simulink model "Dinamica6DOF"  (R2026a)
settings: Solver=FixedStepAuto  StopTime=C.Tfim  FixedStep=0.01  MaxStep=0.001
values from neighbouring files (symbols this model uses):
  C = CondLanc6DOF    [VooUnico6DOF.m]
  cte_grav = 9.8    [CondLanc6DOF.m]    (also in DadosMissil.m; VooUnico6DOF.m; plot6DOF.m)
  D = DadosCGInerciaComum(D)    [DadosCGInercia.m]    (also in PlotGMax.m = DadosCGInercia(D); VooUnico6DOF.m = DadosCGInercia(D))
  dados =     [M_aed.mat]
  M_CD = [8.341 8.24 8.141 8.043 7.946 7.851 7.76 7.674 7.595 7.523 7.46 7.4 ... (1365 elements, 21x5x13)]    [M_aed.mat]
  M_CM = [42.757 43.119 43.498 43.905 44.357 44.839 45.319 45.775 46.191 46.536 46.769 46.963 ... (1365 elements, 21x5x13)]    [M_aed.mat]
  M_CMQ = [-1543.746 -1552.906 -1559.915 -1565.64 -1570.662 -1573.443 -1572.931 -1569.859 -1564.198 -1553.449 -1535.22 -1514.504 ... (1365 elements, 21x5x13)]    [M_aed.mat]
  M_CN = [-21.126 -21.088 -21.046 -20.997 -20.94 -20.877 -20.812 -20.749 -20.692 -20.644 -20.613 -20.587 ... (1365 elements, 21x5x13)]    [M_aed.mat]
  R2D = 180/pi    (= 57.2957795131)    [VooUnico6DOF.m]    (also in plot6DOF.m)
undefined symbols (not defined in the file or in its folder): Newton, Raphson
libraries: aerolibasang x4, sharedutil x2, shared6dof x2, aerolibatmos2 x1, dspmtrx3 x1
settings Model: Creator=carlberto-old  LastModifiedBy=Savio
settings SolverCC: AlgebraicLoopSolver=LineSearch

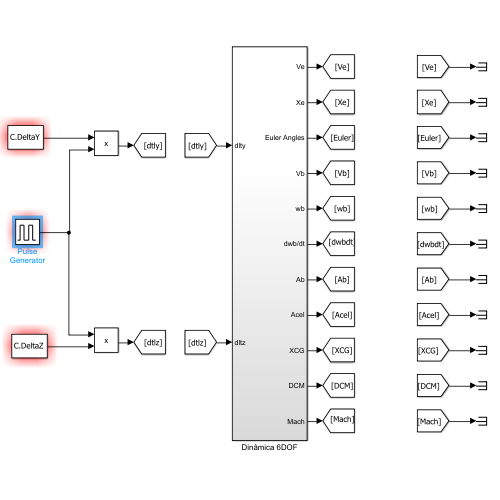
[thumbnail: Simulink's stored preview of the top-level diagram]
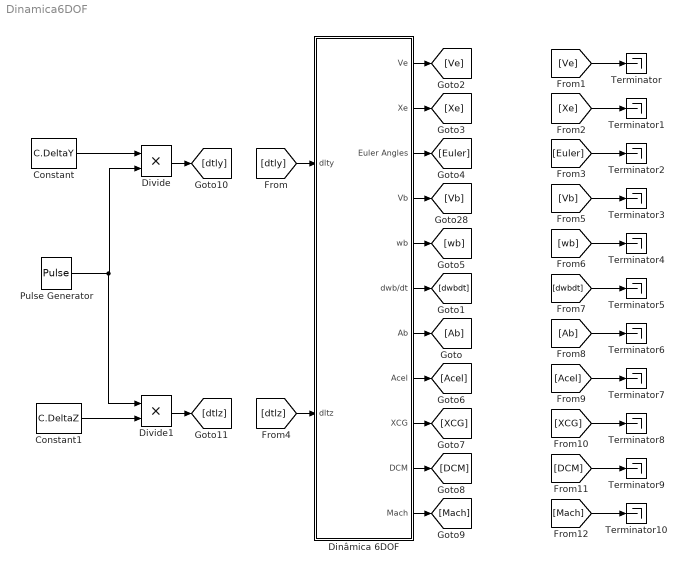
== system Dinamica6DOF ==
  Constant : Constant  Value=C.DeltaY
  Constant1 : Constant  Value=C.DeltaZ
  Dinâmica 6DOF : Subsystem
  Divide : Product  Inputs=**
  Divide1 : Product  Inputs=**
  Pulse Generator : DiscretePulseGenerator  PulseType=Time based  Period=C.Tfim/4  PulseWidth=50  PhaseDelay=D.TTrav
  Terminator{,1..10} (11 alike) : Terminator
  wires:
  Dinâmica 6DOF/2(Xe) -> [Xe]
  Dinâmica 6DOF/3(Euler Angles) -> [Euler]
  Dinâmica 6DOF/5(wb) -> [wb]
  Dinâmica 6DOF/1(Ve) -> [Ve]
  Dinâmica 6DOF/7(Ab) -> [Ab]
  Dinâmica 6DOF/6(dwb/dt) -> [dwbdt]
  Dinâmica 6DOF/4(Vb) -> [Vb]
  Dinâmica 6DOF/10(DCM) -> [DCM]
  Dinâmica 6DOF/9(XCG) -> [XCG]
  Dinâmica 6DOF/8(Acel) -> [Acel]
  Dinâmica 6DOF/11(Mach) -> [Mach]
  [dtlz] -> Dinâmica 6DOF/2(dltz)
  [dtly] -> Dinâmica 6DOF/1(dlty)
  [Ve] -> Terminator/1
  [Xe] -> Terminator1/1
  [Euler] -> Terminator2/1
  [Vb] -> Terminator3/1
  [wb] -> Terminator4/1
  [dwbdt] -> Terminator5/1
  [Ab] -> Terminator6/1
  [Acel] -> Terminator7/1
  [XCG] -> Terminator8/1
  [DCM] -> Terminator9/1
  [Mach] -> Terminator10/1
  Divide/1 -> [dtly]
  Constant/1 -> Divide/1
  Pulse Generator/1 -> Divide1/1, Divide/2
  Divide1/1 -> [dtlz]
  Constant1/1 -> Divide1/2

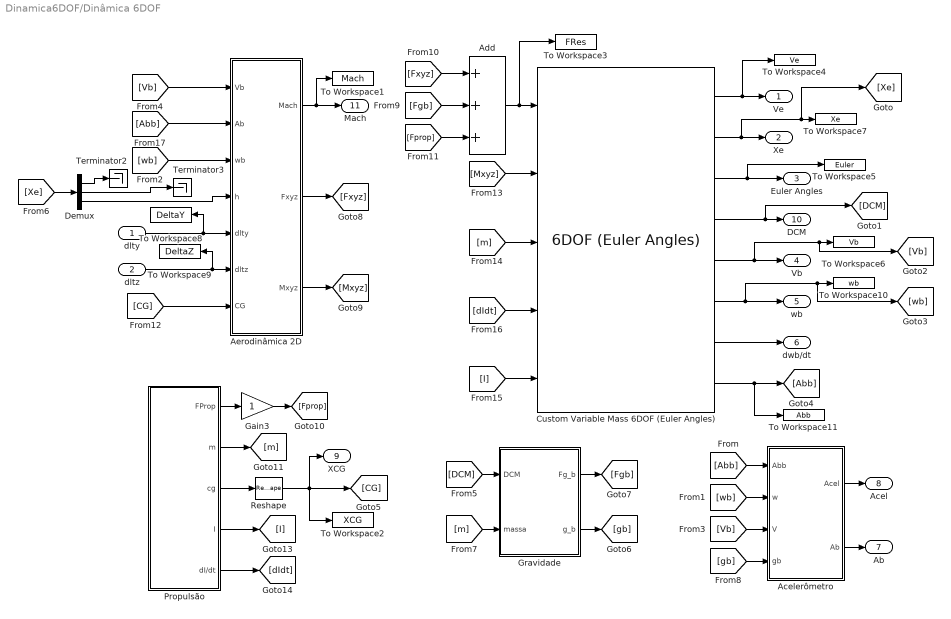
== system Dinamica6DOF/Dinâmica 6DOF ==
  dlty : Inport
  dltz : Inport  Port=2
  Acelerômetro : Subsystem
  Add : Sum  Inputs=+++
  Aerodinâmica 2D : Subsystem
  Custom Variable Mass 6DOF (Euler Angles) : shared6dof/6DOF (Euler Angles)  units=Metric (MKS)  mtype=Custom Variable  rep=Euler Angles  xme_0=[C.Xm0 C.Ym0 -C.Zm0]  Vm_0="[C.Vmx0  C.Vmy0   C.Vmz0]"  eul_0="[C.Phim0  C.Tetam0   C.Psim0]"  pm_0=[C.p0 C.q0 C.r0]  mass_0=1.0  mass_e=0.5  mass_f=2.0  inertia=eye(3)  inertia_e=eye(3)  inertia_f=2*eye(3)  k_quat=1.0  vre_flag=off  abi_flag=off  aMode=aMode  xme_statename=''  Vm_statename=''  eul_statename=''  quat_statename=''  pm_statename=''  mass_statename=''
  Demux : Demux  Outputs=3
  Gain3 : Gain
  Gravidade : Subsystem
  Propulsão : Subsystem
  Reshape : Reshape
  Terminator2 : Terminator
  Terminator3 : Terminator
  To Workspace1 : ToWorkspace  VariableName=Mach  SaveFormat=Timeseries  SampleTime=-1
  To Workspace10 : ToWorkspace  VariableName=wb  SaveFormat=Timeseries  SampleTime=-1
  To Workspace11 : ToWorkspace  VariableName=Abb  SaveFormat=Timeseries  SampleTime=-1
  To Workspace2 : ToWorkspace  VariableName=XCG  SaveFormat=Timeseries  SampleTime=-1
  To Workspace3 : ToWorkspace  VariableName=FRes  SaveFormat=Timeseries  SampleTime=-1
  To Workspace4 : ToWorkspace  VariableName=Ve  SaveFormat=Timeseries  SampleTime=-1
  To Workspace5 : ToWorkspace  VariableName=Euler  SaveFormat=Timeseries  SampleTime=-1
  To Workspace6 : ToWorkspace  VariableName=Vb  SaveFormat=Timeseries  SampleTime=-1
  To Workspace7 : ToWorkspace  VariableName=Xe  SaveFormat=Timeseries  SampleTime=-1
  To Workspace8 : ToWorkspace  VariableName=DeltaY  SaveFormat=Timeseries  SampleTime=-1
  To Workspace9 : ToWorkspace  VariableName=DeltaZ  SaveFormat=Timeseries  SampleTime=-1
  Ve : Outport  VectorParamsAs1DForOutWhenUnconnected=off
  Xe : Outport  Port=2  VectorParamsAs1DForOutWhenUnconnected=off
  Euler Angles : Outport  Port=3  VectorParamsAs1DForOutWhenUnconnected=off
  Vb : Outport  Port=4  VectorParamsAs1DForOutWhenUnconnected=off
  wb : Outport  Port=5  VectorParamsAs1DForOutWhenUnconnected=off
  dwb/dt : Outport  Port=6  VectorParamsAs1DForOutWhenUnconnected=off
  Ab : Outport  Port=7  VectorParamsAs1DForOutWhenUnconnected=off
  Acel : Outport  Port=8  VectorParamsAs1DForOutWhenUnconnected=off
  XCG : Outport  Port=9  VectorParamsAs1DForOutWhenUnconnected=off
  DCM : Outport  Port=10  VectorParamsAs1DForOutWhenUnconnected=off
  Mach : Outport  Port=11  VectorParamsAs1DForOutWhenUnconnected=off
  wires:
  Custom Variable Mass 6DOF (Euler Angles)/1 -> To Workspace4/1, Ve/1
  Custom Variable Mass 6DOF (Euler Angles)/3 -> To Workspace5/1, Euler Angles/1
  Custom Variable Mass 6DOF (Euler Angles)/7 -> dwb/dt/1
  Add/1 -> To Workspace3/1, Custom Variable Mass 6DOF (Euler Angles)/1
  Custom Variable Mass 6DOF (Euler Angles)/4 -> DCM/1, [DCM]
  Reshape/1 -> XCG/1, [CG], To Workspace2/1
  Propulsão/3(cg) -> Reshape/1
  [Abb] -> Acelerômetro/1(Abb)
  [wb] -> Acelerômetro/2(w)
  [Vb] -> Acelerômetro/3(V)
  [DCM] -> Gravidade/1(DCM)
  Acelerômetro/2(Ab) -> Ab/1
  [gb] -> Acelerômetro/4(gb)
  Propulsão/2(m) -> [m]
  Propulsão/4(I) -> [I]
  Propulsão/5(dI/dt) -> [dIdt]
  [m] -> Custom Variable Mass 6DOF (Euler Angles)/3
  [I] -> Custom Variable Mass 6DOF (Euler Angles)/5
  [dIdt] -> Custom Variable Mass 6DOF (Euler Angles)/4
  Custom Variable Mass 6DOF (Euler Angles)/6 -> [wb], To Workspace10/1, wb/1
  Custom Variable Mass 6DOF (Euler Angles)/8 -> [Abb], To Workspace11/1
  Custom Variable Mass 6DOF (Euler Angles)/5 -> To Workspace6/1, [Vb], Vb/1
  [m] -> Gravidade/2(massa)
  [Fxyz] -> Add/1
  Gravidade/1(Fg_b) -> [Fgb]
  [Mxyz] -> Custom Variable Mass 6DOF (Euler Angles)/2
  Acelerômetro/1(Acel) -> Acel/1
  Custom Variable Mass 6DOF (Euler Angles)/2 -> [Xe], To Workspace7/1, Xe/1
  Gravidade/2(g_b) -> [gb]
  [Fgb] -> Add/2
  [Fprop] -> Add/3
  Demux/1 -> Terminator2/1
  [Xe] -> Demux/1
  [CG] -> Aerodinâmica 2D/7(CG)
  dlty/1 -> To Workspace8/1, Aerodinâmica 2D/5(dlty)
  Demux/2 -> Terminator3/1
  Aerodinâmica 2D/1(Mach) -> To Workspace1/1, Mach/1
  Aerodinâmica 2D/3(Mxyz) -> [Mxyz]
  [wb] -> Aerodinâmica 2D/3(wb)
  [Vb] -> Aerodinâmica 2D/1(Vb)
  [Abb] -> Aerodinâmica 2D/2(Ab)
  Aerodinâmica 2D/2(Fxyz) -> [Fxyz]
  Demux/3 -> Aerodinâmica 2D/4(h)
  dltz/1 -> Aerodinâmica 2D/6(dltz), To Workspace9/1
  Propulsão/1(FProp) -> Gain3/1
  Gain3/1 -> [Fprop]

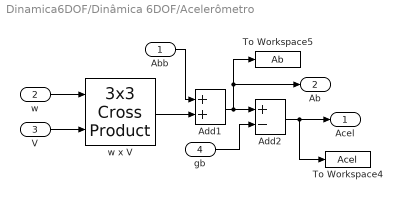
== system Dinamica6DOF/Dinâmica 6DOF/Acelerômetro ==
  Abb : Inport
  w : Inport  Port=2
  V : Inport  Port=3
  gb : Inport  Port=4
  Add1 : Sum
  Add2 : Sum  Inputs=+-
  To Workspace4 : ToWorkspace  VariableName=Acel  SaveFormat=Timeseries  SampleTime=-1
  To Workspace5 : ToWorkspace  VariableName=Ab  SaveFormat=Timeseries  SampleTime=-1
  w x V : sharedutil/3x3 Cross Product  aMode=aMode
  Acel : Outport  VectorParamsAs1DForOutWhenUnconnected=off
  Ab : Outport  Port=2  VectorParamsAs1DForOutWhenUnconnected=off
  wires:
  V/1 -> w x V/2
  w/1 -> w x V/1
  Add1/1 -> Add2/1, Ab/1, To Workspace5/1
  Add2/1 -> To Workspace4/1, Acel/1
  gb/1 -> Add2/2
  w x V/1 -> Add1/2
  Abb/1 -> Add1/1

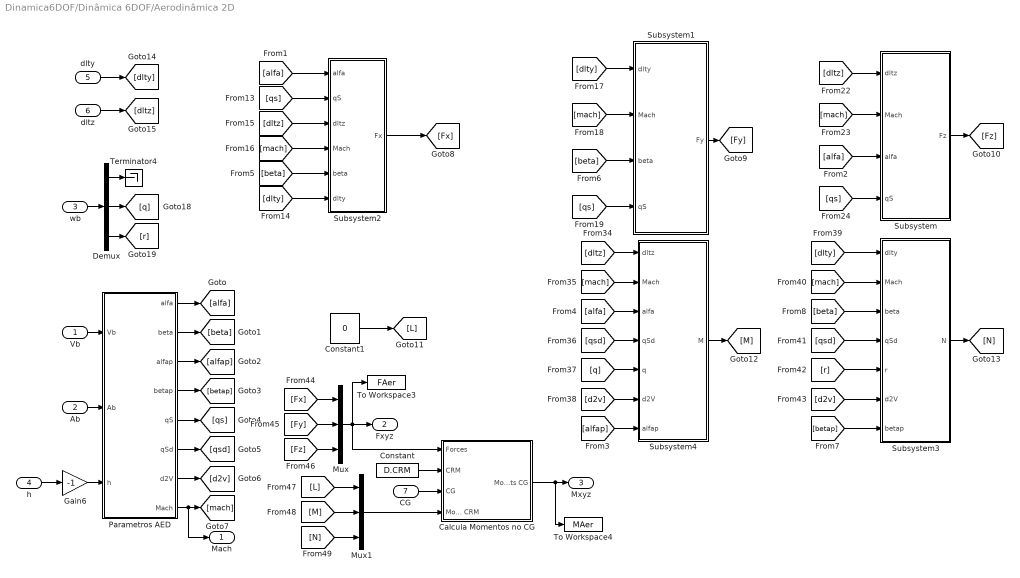
== system Dinamica6DOF/Dinâmica 6DOF/Aerodinâmica 2D ==
  Vb : Inport
  Ab : Inport  Port=2
  wb : Inport  Port=3
  h : Inport  Port=4
  dlty : Inport  Port=5
  dltz : Inport  Port=6
  CG : Inport  Port=7
  Calcula Momentos no CG : Subsystem
  Constant : Constant  Value=D.CRM
  Constant1 : Constant  Value=0
  Demux : Demux  Outputs=3
  Gain6 : Gain  Gain=-1
  Mux : Mux  Inputs=3
  Mux1 : Mux  Inputs=3
  Parametros AED : Subsystem
  Subsystem : Subsystem
  Subsystem1 : Subsystem
  Subsystem2 : Subsystem
  Subsystem3 : Subsystem
  Subsystem4 : Subsystem
  Terminator4 : Terminator
  To Workspace3 : ToWorkspace  VariableName=FAer  SaveFormat=Timeseries  SampleTime=-1
  To Workspace4 : ToWorkspace  VariableName=MAer  SaveFormat=Timeseries  SampleTime=-1
  Mach : Outport  VectorParamsAs1DForOutWhenUnconnected=off
  Fxyz : Outport  Port=2  VectorParamsAs1DForOutWhenUnconnected=off
  Mxyz : Outport  Port=3  VectorParamsAs1DForOutWhenUnconnected=off
  wires:
  h/1 -> Gain6/1
  Mux1/1 -> Calcula Momentos no CG/4(Moments CRM)
  wb/1 -> Demux/1
  Vb/1 -> Parametros AED/1(Vb)
  Ab/1 -> Parametros AED/2(Ab)
  Gain6/1 -> Parametros AED/3(h)
  CG/1 -> Calcula Momentos no CG/3(CG)
  Constant/1 -> Calcula Momentos no CG/2(CRM)
  Calcula Momentos no CG/1(Moments CG) -> To Workspace4/1, Mxyz/1
  Parametros AED/1(alfa) -> [alfa]
  [alfa] -> Subsystem2/1(alfa)
  [alfa] -> Subsystem/3(alfa)
  [alfa] -> Subsystem4/3(alfa)
  Parametros AED/2(beta) -> [beta]
  [beta] -> Subsystem1/3(beta)
  [beta] -> Subsystem3/3(beta)
  Parametros AED/3(alfap) -> [alfap]
  Parametros AED/4(betap) -> [betap]
  Parametros AED/5(qS) -> [qs]
  Parametros AED/6(qSd) -> [qsd]
  Parametros AED/7(d2V) -> [d2v]
  Parametros AED/8(Mach) -> Mach/1, [mach]
  [qs] -> Subsystem2/2(qS)
  [dlty] -> Subsystem2/6(dlty)
  [dltz] -> Subsystem2/3(dltz)
  [mach] -> Subsystem2/4("Mach ")
  [dlty] -> Subsystem1/1("dlty ")
  [mach] -> Subsystem1/2(Mach)
  [qs] -> Subsystem1/4(qS)
  Subsystem1/1(Fy) -> [Fy]
  [dltz] -> Subsystem/1(dltz)
  [mach] -> Subsystem/2("Mach ")
  [qs] -> Subsystem/4(qS)
  Subsystem/1(Fz) -> [Fz]
  [dltz] -> Subsystem4/1(dltz)
  [mach] -> Subsystem4/2(Mach)
  [qsd] -> Subsystem4/4(qSd)
  [q] -> Subsystem4/5(q)
  [d2v] -> Subsystem4/6(d2V)
  Subsystem4/1(M) -> [M]
  [dlty] -> Subsystem3/1(dlty)
  [mach] -> Subsystem3/2(Mach)
  [qsd] -> Subsystem3/4(qSd)
  [r] -> Subsystem3/5(r)
  [d2v] -> Subsystem3/6(d2V)
  Subsystem3/1(N) -> [N]
  [Fx] -> Mux/1
  [Fy] -> Mux/2
  [Fz] -> Mux/3
  [L] -> Mux1/1
  [M] -> Mux1/2
  [N] -> Mux1/3
  dlty/1 -> [dlty]
  dltz/1 -> [dltz]
  Demux/1 -> Terminator4/1
  Demux/2 -> [q]
  Demux/3 -> [r]
  Constant1/1 -> [L]
  [beta] -> Subsystem2/5(beta)
  [alfap] -> Subsystem4/7(alfap)
  [betap] -> Subsystem3/7(betap)
  Subsystem2/1(Fx) -> [Fx]
  Mux/1 -> Calcula Momentos no CG/1(Forces), Fxyz/1, To Workspace3/1

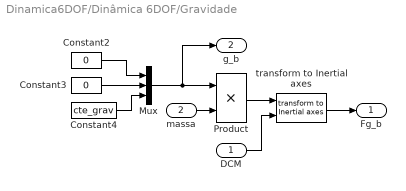
== system Dinamica6DOF/Dinâmica 6DOF/Gravidade ==
  DCM : Inport
  massa : Inport  Port=2
  Constant2 : Constant  Value=0
  Constant3 : Constant  Value=0
  Constant4 : Constant  Value=cte_grav
  Mux : Mux  Inputs=3
  Product : Product
  "transform to Inertial axes " : shared6dof/6DOF (Euler Angles)/transform to Inertial axes   SystemSampleTime=-1
      settings: SourceProductName=Aerospace Blockset
  Fg_b : Outport  VectorParamsAs1DForOutWhenUnconnected=off
  g_b : Outport  Port=2  VectorParamsAs1DForOutWhenUnconnected=off
  wires:
  Constant3/1 -> Mux/2
  Constant2/1 -> Mux/1
  Constant4/1 -> Mux/3
  Mux/1 -> g_b/1, Product/1
  DCM/1 -> "transform to Inertial axes "/2
  "transform to Inertial axes "/1 -> Fg_b/1
  Product/1 -> "transform to Inertial axes "/1
  massa/1 -> Product/2

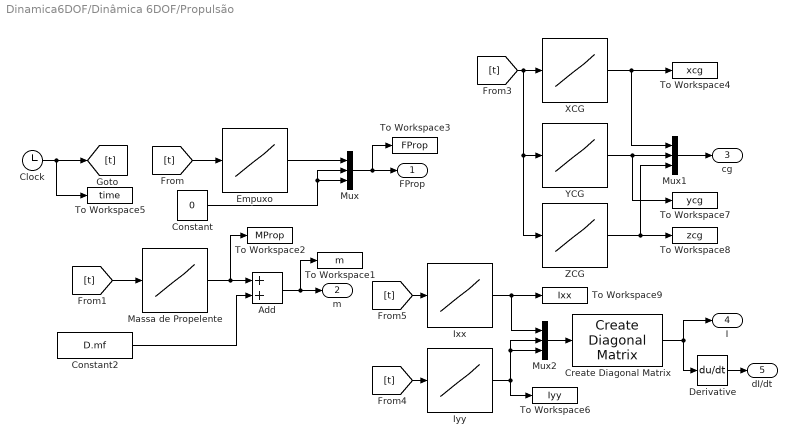
== system Dinamica6DOF/Dinâmica 6DOF/Propulsão ==
  Add : Sum
  Clock : Clock
  Constant : Constant  Value=0
  Constant2 : Constant  Value=D.mf
  Create Diagonal Matrix : dspmtrx3/Create Diagonal Matrix
      settings: SourceProductName=DSP System Toolbox
  Derivative : Derivative
  "Empuxo " : Lookup_n-D  NumberOfTableDimensions=1  BreakpointsForDimension1=D.VProp(:,1)  Table=D.VProp(:,2)  ExtrapMethod=Clip  InternalRulePriority=Speed  RndMeth=Simplest
  Ixx : Lookup_n-D  NumberOfTableDimensions=1  BreakpointsForDimension1=D.IMissil(:,1)  Table=D.IMissil(:,2)  ExtrapMethod=Clip  InternalRulePriority=Speed  RndMeth=Simplest
  Iyy : Lookup_n-D  NumberOfTableDimensions=1  BreakpointsForDimension1=D.IMissil(:,1)  Table=D.IMissil(:,3)  ExtrapMethod=Clip  InternalRulePriority=Speed  RndMeth=Simplest
  Massa de Propelente : Lookup_n-D  NumberOfTableDimensions=1  BreakpointsForDimension1=D.VProp(:,1)  Table=D.VProp(:,3)  ExtrapMethod=Clip  InternalRulePriority=Speed  RndMeth=Simplest
  Mux : Mux  Inputs=3
  Mux1 : Mux  Inputs=3
  Mux2 : Mux  Inputs=3
  To Workspace1 : ToWorkspace  VariableName=m  SaveFormat=Timeseries  SampleTime=-1
  To Workspace2 : ToWorkspace  VariableName=MProp  SaveFormat=Timeseries  SampleTime=-1
  To Workspace3 : ToWorkspace  VariableName=FProp  SaveFormat=Timeseries  SampleTime=-1
  To Workspace4 : ToWorkspace  VariableName=xcg  SaveFormat=Timeseries  SampleTime=-1
  To Workspace5 : ToWorkspace  VariableName=time  SaveFormat=Timeseries  SampleTime=-1
  To Workspace6 : ToWorkspace  VariableName=Iyy  SaveFormat=Timeseries  SampleTime=-1
  To Workspace7 : ToWorkspace  VariableName=ycg  SaveFormat=Timeseries  SampleTime=-1
  To Workspace8 : ToWorkspace  VariableName=zcg  SaveFormat=Timeseries  SampleTime=-1
  To Workspace9 : ToWorkspace  VariableName=Ixx  SaveFormat=Timeseries  SampleTime=-1
  "XCG " : Lookup_n-D  NumberOfTableDimensions=1  BreakpointsForDimension1=D.CGMissil(:,1)  Table=D.CGMissil(:,2)  ExtrapMethod=Clip  InternalRulePriority=Speed  RndMeth=Simplest
  "YCG " : Lookup_n-D  NumberOfTableDimensions=1  BreakpointsForDimension1=D.CGMissil(:,1)  Table=D.CGMissil(:,3)  ExtrapMethod=Clip  InternalRulePriority=Speed  RndMeth=Simplest
  "ZCG " : Lookup_n-D  NumberOfTableDimensions=1  BreakpointsForDimension1=D.CGMissil(:,1)  Table=D.CGMissil(:,4)  ExtrapMethod=Clip  InternalRulePriority=Speed  RndMeth=Simplest
  FProp : Outport  VectorParamsAs1DForOutWhenUnconnected=off
  m : Outport  Port=2  VectorParamsAs1DForOutWhenUnconnected=off
  cg : Outport  Port=3  VectorParamsAs1DForOutWhenUnconnected=off
  I : Outport  Port=4  VectorParamsAs1DForOutWhenUnconnected=off
  dI/dt : Outport  Port=5  VectorParamsAs1DForOutWhenUnconnected=off
  wires:
  Mux/1 -> FProp/1, To Workspace3/1
  "Empuxo "/1 -> Mux/1
  Constant/1 -> Mux/3, Mux/2
  Massa de Propelente/1 -> To Workspace2/1, Add/1
  Add/1 -> m/1, To Workspace1/1
  Constant2/1 -> Add/2
  Derivative/1 -> dI/dt/1
  Mux1/1 -> cg/1
  "XCG "/1 -> To Workspace4/1, Mux1/1
  Create Diagonal Matrix/1 -> I/1, Derivative/1
  Ixx/1 -> To Workspace9/1, Mux2/1
  Iyy/1 -> To Workspace6/1, Mux2/3, Mux2/2
  Mux2/1 -> Create Diagonal Matrix/1
  [t] -> "Empuxo "/1
  [t] -> Massa de Propelente/1
  [t] -> "ZCG "/1, "YCG "/1, "XCG "/1
  [t] -> Ixx/1
  [t] -> Iyy/1
  "YCG "/1 -> To Workspace7/1, Mux1/2
  "ZCG "/1 -> Mux1/3, To Workspace8/1
  Clock/1 -> To Workspace5/1, [t]

== system Dinamica6DOF/Dinâmica 6DOF/Aerodinâmica 2D/Calcula Momentos no CG ==
  Forces : Inport
  CRM : Inport  Port=2
  CG : Inport  Port=3
  Moments CRM : Inport  Port=4
  3x3 Cross Product : sharedutil/3x3 Cross Product  aMode=aMode
  Sum : Sum  Inputs=|+-  SaturateOnIntegerOverflow=on
  Sum1 : Sum  Inputs=|++  SaturateOnIntegerOverflow=on
  To Workspace : ToWorkspace  VariableName=Delta_CG  SaveFormat=Timeseries  SampleTime=-1
  Moments CG : Outport  VectorParamsAs1DForOutWhenUnconnected=off
  wires:
  CRM/1 -> Sum/1
  CG/1 -> Sum/2
  Sum/1 -> 3x3 Cross Product/1, To Workspace/1
  Forces/1 -> 3x3 Cross Product/2
  Moments CRM/1 -> Sum1/2
  Sum1/1 -> Moments CG/1
  3x3 Cross Product/1 -> Sum1/1

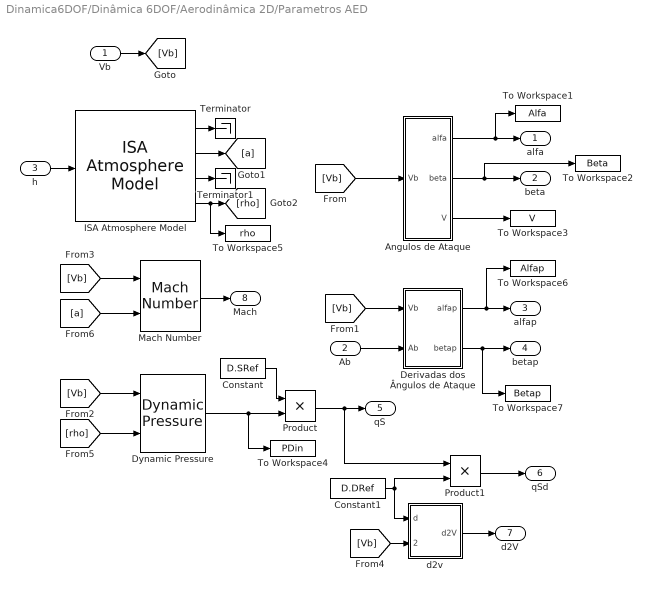
== system Dinamica6DOF/Dinâmica 6DOF/Aerodinâmica 2D/Parametros AED ==
  Vb : Inport
  Ab : Inport  Port=2
  h : Inport  Port=3
  Angulos de Ataque : Subsystem
  Constant : Constant  Value=D.SRef
  Constant1 : Constant  Value=D.DRef
  Derivadas dos Ângulos de Ataque : Subsystem
  Dynamic Pressure : aerolibasang/Dynamic Pressure
  ISA Atmosphere Model : aerolibatmos2/ISA Atmosphere Model  custom=off  g=9.80665  gamma=1.4  R=287.0531  L=0.0065  h_trop=11000  h_strat=20000  rho0=1.225  P0=101325  T0=288.15  h0=0
      settings: SourceProductName=Aerospace Blockset
  Mach Number : aerolibasang/Mach Number
      settings: SourceProductName=Aerospace Blockset
  Product : Product
  Product1 : Product
  Terminator : Terminator
  Terminator1 : Terminator
  To Workspace1 : ToWorkspace  VariableName=Alfa  SaveFormat=Timeseries  SampleTime=-1
  To Workspace2 : ToWorkspace  VariableName=Beta  SaveFormat=Timeseries  SampleTime=-1
  To Workspace3 : ToWorkspace  VariableName=V  SaveFormat=Timeseries  SampleTime=-1
  To Workspace4 : ToWorkspace  VariableName=PDin  SaveFormat=Timeseries  SampleTime=-1
  To Workspace5 : ToWorkspace  VariableName=rho  SaveFormat=Timeseries  SampleTime=-1
  To Workspace6 : ToWorkspace  VariableName=Alfap  SaveFormat=Timeseries  SampleTime=-1
  To Workspace7 : ToWorkspace  VariableName=Betap  SaveFormat=Timeseries  SampleTime=-1
  d2v : Subsystem
  alfa : Outport  VectorParamsAs1DForOutWhenUnconnected=off
  beta : Outport  Port=2  VectorParamsAs1DForOutWhenUnconnected=off
  alfap : Outport  Port=3  VectorParamsAs1DForOutWhenUnconnected=off
  betap : Outport  Port=4  VectorParamsAs1DForOutWhenUnconnected=off
  qS : Outport  Port=5  VectorParamsAs1DForOutWhenUnconnected=off
  qSd : Outport  Port=6  VectorParamsAs1DForOutWhenUnconnected=off
  d2V : Outport  Port=7  VectorParamsAs1DForOutWhenUnconnected=off
  Mach : Outport  Port=8  VectorParamsAs1DForOutWhenUnconnected=off
  wires:
  Derivadas dos Ângulos de Ataque/2(betap) -> To Workspace7/1, betap/1
  Derivadas dos Ângulos de Ataque/1(alfap) -> To Workspace6/1, alfap/1
  h/1 -> ISA Atmosphere Model/1
  Constant/1 -> Product/1
  Dynamic Pressure/1 -> To Workspace4/1, Product/2
  ISA Atmosphere Model/4 -> To Workspace5/1, [rho]
  Constant1/1 -> Product1/2, d2v/1(d)
  Product1/1 -> qSd/1
  d2v/1(d2V) -> d2V/1
  Product/1 -> Product1/1, qS/1
  Angulos de Ataque/3(V) -> To Workspace3/1
  Angulos de Ataque/1(alfa) -> To Workspace1/1, alfa/1
  Angulos de Ataque/2(beta) -> beta/1, To Workspace2/1
  Mach Number/1 -> Mach/1
  Vb/1 -> [Vb]
  [Vb] -> Angulos de Ataque/1(Vb)
  [Vb] -> Derivadas dos Ângulos de Ataque/1(Vb)
  [Vb] -> Dynamic Pressure/1
  [Vb] -> Mach Number/1
  [Vb] -> d2v/2(Velocity)
  [rho] -> Dynamic Pressure/2
  [a] -> Mach Number/2
  ISA Atmosphere Model/2 -> [a]
  ISA Atmosphere Model/1 -> Terminator/1
  ISA Atmosphere Model/3 -> Terminator1/1
  Ab/1 -> Derivadas dos Ângulos de Ataque/2(Ab)

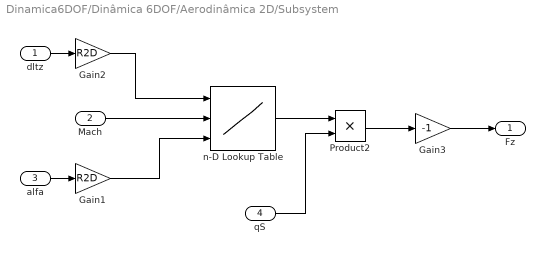
== system Dinamica6DOF/Dinâmica 6DOF/Aerodinâmica 2D/Subsystem ==
  dltz : Inport
  "Mach " : Inport  Port=2
  alfa : Inport  Port=3
  qS : Inport  Port=4
  Gain1 : Gain  Gain=R2D
  Gain2 : Gain  Gain=R2D
  Gain3 : Gain  Gain=-1
  Product2 : Product
  n-D Lookup Table : Lookup_n-D  NumberOfTableDimensions=3  BreakpointsForDimension1=dados.delta  BreakpointsForDimension2=dados.mach  BreakpointsForDimension3=dados.alpha  Table=M_CN  ExtrapMethod=Clip  InternalRulePriority=Speed  RndMeth=Simplest
      settings: InputPortMap=u0,u1,u2
  Fz : Outport  VectorParamsAs1DForOutWhenUnconnected=off
  wires:
  "Mach "/1 -> n-D Lookup Table/2
  dltz/1 -> Gain2/1
  alfa/1 -> Gain1/1
  Product2/1 -> Gain3/1
  n-D Lookup Table/1 -> Product2/1
  qS/1 -> Product2/2
  Gain2/1 -> n-D Lookup Table/1
  Gain1/1 -> n-D Lookup Table/3
  Gain3/1 -> Fz/1

== system Dinamica6DOF/Dinâmica 6DOF/Aerodinâmica 2D/Subsystem1 ==
  "dlty " : Inport
  Mach : Inport  Port=2
  beta : Inport  Port=3
  qS : Inport  Port=4
  Gain2 : Gain  Gain=-R2D
  Gain3 : Gain  Gain=R2D
  Product1 : Product
  n-D Lookup Table : Lookup_n-D  NumberOfTableDimensions=3  BreakpointsForDimension1=dados.delta  BreakpointsForDimension2=dados.mach  BreakpointsForDimension3=dados.alpha  Table=M_CN  ExtrapMethod=Clip  InternalRulePriority=Speed  RndMeth=Simplest
      settings: InputPortMap=u0,u1,u2
  Fy : Outport  VectorParamsAs1DForOutWhenUnconnected=off
  wires:
  n-D Lookup Table/1 -> Product1/1
  beta/1 -> Gain2/1
  "dlty "/1 -> Gain3/1
  Mach/1 -> n-D Lookup Table/2
  qS/1 -> Product1/2
  Gain3/1 -> n-D Lookup Table/1
  Gain2/1 -> n-D Lookup Table/3
  Product1/1 -> Fy/1

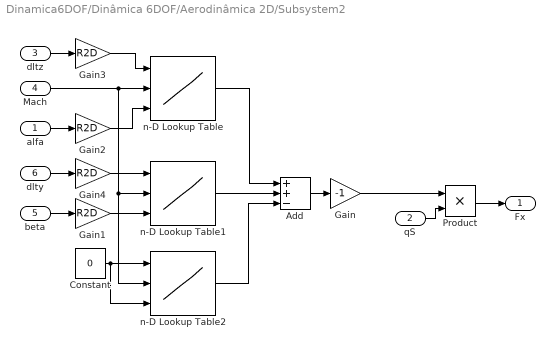
== system Dinamica6DOF/Dinâmica 6DOF/Aerodinâmica 2D/Subsystem2 ==
  alfa : Inport
  qS : Inport  Port=2
  dltz : Inport  Port=3
  "Mach " : Inport  Port=4
  beta : Inport  Port=5
  dlty : Inport  Port=6
  Add : Sum  Inputs=++-
  Constant : Constant  Value=0
  Gain : Gain  Gain=-1
  Gain{1..4} (4 alike) : Gain  Gain=R2D
  Product : Product
  n-D Lookup Table : Lookup_n-D  NumberOfTableDimensions=3  BreakpointsForDimension1=dados.delta  BreakpointsForDimension2=dados.mach  BreakpointsForDimension3=dados.alpha  Table=M_CD  ExtrapMethod=Clip  InternalRulePriority=Speed  RndMeth=Simplest
      settings: InputPortMap=u0,u1,u2
  n-D Lookup Table1 : Lookup_n-D  NumberOfTableDimensions=3  BreakpointsForDimension1=dados.delta  BreakpointsForDimension2=dados.mach  BreakpointsForDimension3=dados.alpha  Table=M_CD  ExtrapMethod=Clip  InternalRulePriority=Speed  RndMeth=Simplest
      settings: InputPortMap=u0,u1,u2
  n-D Lookup Table2 : Lookup_n-D  NumberOfTableDimensions=3  BreakpointsForDimension1=dados.delta  BreakpointsForDimension2=dados.mach  BreakpointsForDimension3=dados.alpha  Table=M_CD  ExtrapMethod=Clip  InternalRulePriority=Speed  RndMeth=Simplest
      settings: InputPortMap=u0,u1,u2
  Fx : Outport  VectorParamsAs1DForOutWhenUnconnected=off
  wires:
  qS/1 -> Product/2
  Gain3/1 -> n-D Lookup Table/1
  Gain2/1 -> n-D Lookup Table/3
  Product/1 -> Fx/1
  Gain1/1 -> n-D Lookup Table1/3
  Gain4/1 -> n-D Lookup Table1/1
  Constant/1 -> n-D Lookup Table2/3, n-D Lookup Table2/1
  n-D Lookup Table2/1 -> Add/3
  "Mach "/1 -> n-D Lookup Table2/2, n-D Lookup Table1/2, n-D Lookup Table/2
  n-D Lookup Table/1 -> Add/1
  n-D Lookup Table1/1 -> Add/2
  Add/1 -> Gain/1
  dltz/1 -> Gain3/1
  alfa/1 -> Gain2/1
  dlty/1 -> Gain4/1
  beta/1 -> Gain1/1
  Gain/1 -> Product/1

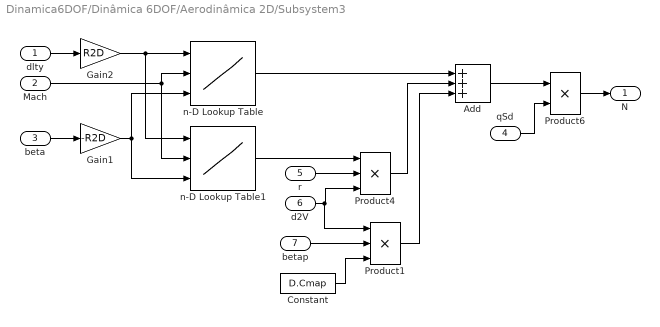
== system Dinamica6DOF/Dinâmica 6DOF/Aerodinâmica 2D/Subsystem3 ==
  dlty : Inport
  Mach : Inport  Port=2
  beta : Inport  Port=3
  qSd : Inport  Port=4
  r : Inport  Port=5
  d2V : Inport  Port=6
  betap : Inport  Port=7
  Add : Sum  Inputs=+++
  Constant : Constant  Value=D.Cmap
  Gain1 : Gain  Gain=-R2D
  Gain2 : Gain  Gain=R2D
  Product1 : Product  Inputs=3
  Product4 : Product  Inputs=3
  Product6 : Product
  n-D Lookup Table : Lookup_n-D  NumberOfTableDimensions=3  BreakpointsForDimension1=dados.delta  BreakpointsForDimension2=dados.mach  BreakpointsForDimension3=dados.alpha  Table=M_CM  ExtrapMethod=Clip  InternalRulePriority=Speed  RndMeth=Simplest
      settings: InputPortMap=u0,u1,u2
  n-D Lookup Table1 : Lookup_n-D  NumberOfTableDimensions=3  BreakpointsForDimension1=dados.delta  BreakpointsForDimension2=dados.mach  BreakpointsForDimension3=dados.alpha  Table=M_CMQ  ExtrapMethod=Clip  InternalRulePriority=Speed  RndMeth=Simplest
      settings: InputPortMap=u0,u1,u2
  N : Outport  VectorParamsAs1DForOutWhenUnconnected=off
  wires:
  d2V/1 -> Product1/1, Product4/3
  Product6/1 -> N/1
  Add/1 -> Product6/1
  qSd/1 -> Product6/2
  r/1 -> Product4/2
  dlty/1 -> Gain2/1
  Mach/1 -> n-D Lookup Table1/2, n-D Lookup Table/2
  beta/1 -> Gain1/1
  Product4/1 -> Add/2
  Gain2/1 -> n-D Lookup Table/1, n-D Lookup Table1/1
  Gain1/1 -> n-D Lookup Table/3, n-D Lookup Table1/3
  n-D Lookup Table/1 -> Add/1
  n-D Lookup Table1/1 -> Product4/1
  Constant/1 -> Product1/3
  Product1/1 -> Add/3
  betap/1 -> Product1/2

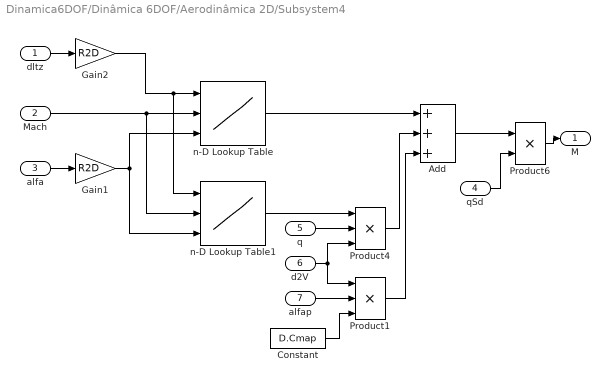
== system Dinamica6DOF/Dinâmica 6DOF/Aerodinâmica 2D/Subsystem4 ==
  dltz : Inport
  Mach : Inport  Port=2
  alfa : Inport  Port=3
  qSd : Inport  Port=4
  q : Inport  Port=5
  d2V : Inport  Port=6
  alfap : Inport  Port=7
  Add : Sum  Inputs=+++
  Constant : Constant  Value=D.Cmap
  Gain1 : Gain  Gain=R2D
  Gain2 : Gain  Gain=R2D
  Product1 : Product  Inputs=3
  Product4 : Product  Inputs=3
  Product6 : Product
  n-D Lookup Table : Lookup_n-D  NumberOfTableDimensions=3  BreakpointsForDimension1=dados.delta  BreakpointsForDimension2=dados.mach  BreakpointsForDimension3=dados.alpha  Table=M_CM  ExtrapMethod=Clip  InternalRulePriority=Speed  RndMeth=Simplest
      settings: InputPortMap=u0,u1,u2
  n-D Lookup Table1 : Lookup_n-D  NumberOfTableDimensions=3  BreakpointsForDimension1=dados.delta  BreakpointsForDimension2=dados.mach  BreakpointsForDimension3=dados.alpha  Table=M_CMQ  ExtrapMethod=Clip  InternalRulePriority=Speed  RndMeth=Simplest
      settings: InputPortMap=u0,u1,u2
  M : Outport  VectorParamsAs1DForOutWhenUnconnected=off
  wires:
  d2V/1 -> Product1/1, Product4/3
  Product6/1 -> M/1
  Add/1 -> Product6/1
  qSd/1 -> Product6/2
  q/1 -> Product4/2
  dltz/1 -> Gain2/1
  alfa/1 -> Gain1/1
  Product4/1 -> Add/2
  Gain2/1 -> n-D Lookup Table1/1, n-D Lookup Table/1
  Gain1/1 -> n-D Lookup Table/3, n-D Lookup Table1/3
  n-D Lookup Table/1 -> Add/1
  n-D Lookup Table1/1 -> Product4/1
  Mach/1 -> n-D Lookup Table/2, n-D Lookup Table1/2
  alfap/1 -> Product1/2
  Product1/1 -> Add/3
  Constant/1 -> Product1/3

== system Dinamica6DOF/Dinâmica 6DOF/Aerodinâmica 2D/Parametros AED/Angulos de Ataque ==
  Vb : Inport
  Airspeed : Sqrt  AlgorithmType=Newton-Raphson
  Demux1 : Demux  Outputs=3
      settings: DisplayOption=none
  Incidence : Trigonometry  Operator=atan2
  Incidence1 : Trigonometry  Operator=atan2
  dot : aerolibasang/Incidence, Sideslip, & Airspeed/dot  SystemSampleTime=-1
      settings: SourceProductName=Aerospace Blockset
  alfa : Outport  VectorParamsAs1DForOutWhenUnconnected=off
  beta : Outport  Port=2  VectorParamsAs1DForOutWhenUnconnected=off
  V : Outport  Port=3  VectorParamsAs1DForOutWhenUnconnected=off
  wires:
  Demux1/3 -> Incidence/1
  Incidence/1 -> alfa/1
  Vb/1 -> Demux1/1, dot/1
  Demux1/2 -> Incidence1/1
  dot/1 -> Airspeed/1
  Airspeed/1 -> V/1
  Incidence1/1 -> beta/1
  Demux1/1 -> Incidence/2, Incidence1/2

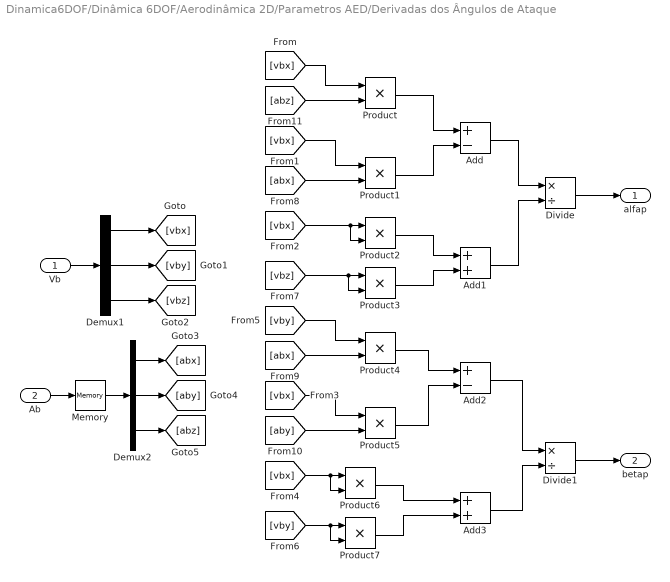
== system Dinamica6DOF/Dinâmica 6DOF/Aerodinâmica 2D/Parametros AED/Derivadas dos Ângulos de Ataque ==
  Vb : Inport
  Ab : Inport  Port=2
  Add : Sum  Inputs=+-
  Add1 : Sum
  Add2 : Sum  Inputs=+-
  Add3 : Sum
  Demux1 : Demux  Outputs=3
  Demux2 : Demux  Outputs=3
  Divide : Product  Inputs=*/
  Divide1 : Product  Inputs=*/
  Memory : Memory
  Product{,1..7} (8 alike) : Product
  alfap : Outport  VectorParamsAs1DForOutWhenUnconnected=off
  betap : Outport  Port=2  VectorParamsAs1DForOutWhenUnconnected=off
  wires:
  Product/1 -> Add/1
  Product1/1 -> Add/2
  Product2/1 -> Add1/1
  Product3/1 -> Add1/2
  Add/1 -> Divide/1
  Add1/1 -> Divide/2
  Divide/1 -> alfap/1
  Product4/1 -> Add2/1
  Divide1/1 -> betap/1
  Product7/1 -> Add3/2
  Add2/1 -> Divide1/1
  Product6/1 -> Add3/1
  Product5/1 -> Add2/2
  Add3/1 -> Divide1/2
  Vb/1 -> Demux1/1
  Demux1/1 -> [vbx]
  Demux1/2 -> [vby]
  Demux1/3 -> [vbz]
  [vbx] -> Product/1
  [vbx] -> Product1/1
  [vbx] -> Product2/2, Product2/1
  [vbx] -> Product5/1
  [vbx] -> Product6/2, Product6/1
  [vby] -> Product4/1
  [vby] -> Product7/2, Product7/1
  [vbz] -> Product3/2, Product3/1
  Memory/1 -> Demux2/1
  Ab/1 -> Memory/1
  Demux2/1 -> [abx]
  Demux2/2 -> [aby]
  Demux2/3 -> [abz]
  [abx] -> Product1/2
  [abx] -> Product4/2
  [aby] -> Product5/2
  [abz] -> Product/2

== system Dinamica6DOF/Dinâmica 6DOF/Aerodinâmica 2D/Parametros AED/d2v ==
  d : Inport
  Velocity : Inport  Port=2
  Divide : Product  Inputs=*/
  d/(2V) : Gain  Gain=1/2  SaturateOnIntegerOverflow=on  OutDataTypeStr=Inherit: Same as input  ParamDataTypeStr=Inherit: Same as input
  dot : aerolibasang/Dynamic Pressure/dot  SystemSampleTime=-1
      settings: SourceProductName=Aerospace Blockset
  vt : Sqrt  AlgorithmType=Newton-Raphson
  d2V : Outport  InitialOutput=0  VectorParamsAs1DForOutWhenUnconnected=off
  wires:
  d/(2V)/1 -> d2V/1
  Velocity/1 -> dot/1
  Divide/1 -> d/(2V)/1
  dot/1 -> vt/1
  d/1 -> Divide/1
  vt/1 -> Divide/2
